simulink model "rotor_dynamics"  (R2023b)
settings: Solver=FixedStepAuto  StartTime=0.0  StopTime=10.0  FixedStep=1e-3  RelTol=1e-3
settings Model: Creator=admin  LastModifiedBy=admin

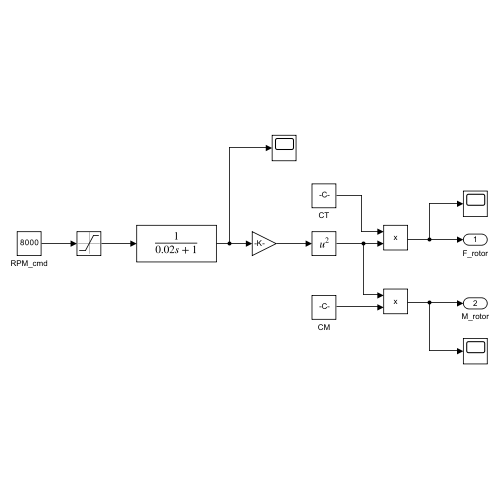
[thumbnail: Simulink's stored preview of the top-level diagram]
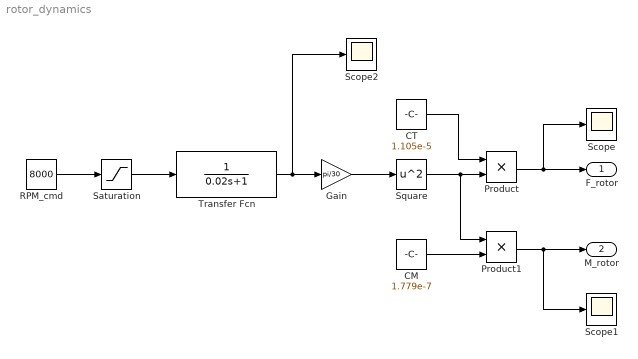
== system rotor_dynamics ==
  CM : Constant  Value=1.779e-7
  CT : Constant  Value=1.105e-5
  Gain : Gain  Gain=pi/30
  Product : Product
  Product1 : Product
  RPM_cmd : Constant  Value=8000
  Saturation : Saturate  UpperLimit=10000  LowerLimit=200
  Scope : Scope
  Scope1 : Scope
  Scope2 : Scope
  Square : Math  Operator=square
  Transfer Fcn : TransferFcn  Denominator=[0.02 1]
  F_rotor : Outport
  M_rotor : Outport  Port=2
  wires:
  RPM_cmd/1 -> Saturation/1
  Saturation/1 -> Transfer Fcn/1
  Transfer Fcn/1 -> Scope2/1, Gain/1
  Gain/1 -> Square/1
  Square/1 -> Product1/1, Product/2
  CT/1 -> Product/1
  CM/1 -> Product1/2
  Product/1 -> Scope/1, F_rotor/1
  Product1/1 -> Scope1/1, M_rotor/1
